simulink library "pidActiveLoad_lib"  (R2013a)
settings: Solver=ode45  StartTime=0.0  StopTime=10.0  RelTol=1e-3
undefined symbols (not defined in the file): dqActiveLoad, dqActiveLoad_lib, Ts
libraries: powerlib x8, simulink x3, breaker_lib x1, Load_lib x1, powerlib_meascontrol x1
settings Model: Creator=ed12083  LastModifiedBy=ed12083

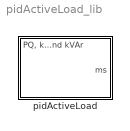
== system pidActiveLoad_lib ==
  pidActiveLoad : Subsystem  AncestorBlock=dqActiveLoad_lib/dqActiveLoad  mask{V=460}
      mask prompts: V "Vbus_RMS"

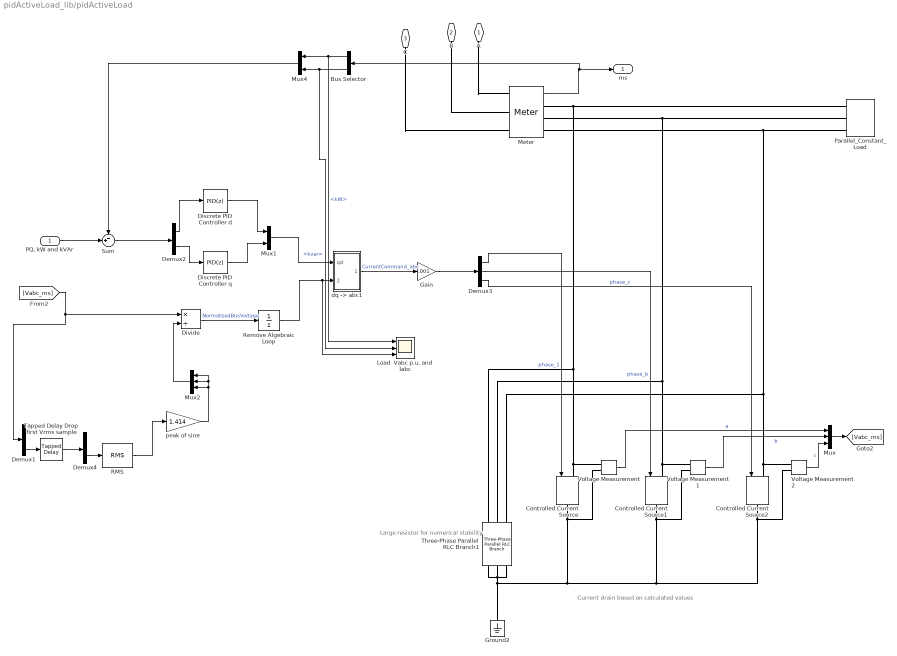
== system pidActiveLoad_lib/pidActiveLoad ==
  note: Current drain based on calculated values
  note: Large resistor for numerical stability
  "PQ, kW and kVAr" : Inport
  Bus Selector : BusSelector  OutputSignals=kW,kvar
  Controlled Current Source : powerlib/Electrical Sources/Controlled Current Source  Initialize=on  Source_Type=AC  Amplitude=0  Phase=0  Frequency=0  Measurements=None
  Controlled Current Source1 : powerlib/Electrical Sources/Controlled Current Source  Initialize=on  Source_Type=AC  Amplitude=0  Phase=0  Frequency=0  Measurements=None
  Controlled Current Source2 : powerlib/Electrical Sources/Controlled Current Source  Initialize=on  Source_Type=AC  Amplitude=0  Phase=0  Frequency=0  Measurements=None
  Demux1 : Demux  Outputs=3
  Demux2 : Demux  Outputs=2
  Demux3 : Demux  Outputs=3
  Demux4 : Demux  Outputs=2
  Discrete PID Controller d : simulink/Continuous/PID Controller  Controller=PID  TimeDomain=Discrete-time  SampleTime=Ts  IntegratorMethod=Forward Euler  FilterMethod=Forward Euler  Form=Parallel  P=0  I=2000  D=20  N=100  InitialConditionSource=internal  InitialConditionForIntegrator=0  InitialConditionForFilter=0  ExternalReset=none  LimitOutput=off  UpperSaturationLimit=inf  LowerSaturationLimit=-inf  LinearizeAsGain=off  AntiWindupMode=none  Kb=1  TrackingMode=off  Kt=1  PParamMin=[]  PParamMax=[]  IParamMin=[]  IParamMax=[]  DParamMin=[]  DParamMax=[]  NParamMin=[]  NParamMax=[]  KbParamMin=[]  KbParamMax=[]  KtParamMin=[]  KtParamMax=[]  POutMin=[]  POutMax=[]  IOutMin=[]  IOutMax=[]  DOutMin=[]  DOutMax=[]  NOutMin=[]  NOutMax=[]  KbOutMin=[]  KbOutMax=[]  KtOutMin=[]  KtOutMax=[]  IntegratorOutMin=[]  IntegratorOutMax=[]  FilterOutMin=[]  FilterOutMax=[]  SumOutMin=[]  SumOutMax=[]  SumI1OutMin=[]  SumI1OutMax=[]  SumI2OutMin=[]  SumI2OutMax=[]  SumI3OutMin=[]  SumI3OutMax=[]  SumDOutMin=[]  SumDOutMax=[]  SaturationOutMin=[]  SaturationOutMax=[]  IntegratorContinuousStateAttributes=''  IntegratorStateMustResolveToSignalObject=off  IntegratorRTWStateStorageClass=Auto  FilterContinuousStateAttributes=''  FilterStateMustResolveToSignalObject=off  FilterRTWStateStorageClass=Auto
  Discrete PID Controller q : simulink/Continuous/PID Controller  Controller=PID  TimeDomain=Discrete-time  SampleTime=Ts  IntegratorMethod=Forward Euler  FilterMethod=Forward Euler  Form=Parallel  P=0  I=-2000  D=-20  N=100  InitialConditionSource=internal  InitialConditionForIntegrator=0  InitialConditionForFilter=0  ExternalReset=none  LimitOutput=off  UpperSaturationLimit=inf  LowerSaturationLimit=-inf  LinearizeAsGain=off  AntiWindupMode=none  Kb=1  TrackingMode=off  Kt=1  PParamMin=[]  PParamMax=[]  IParamMin=[]  IParamMax=[]  DParamMin=[]  DParamMax=[]  NParamMin=[]  NParamMax=[]  KbParamMin=[]  KbParamMax=[]  KtParamMin=[]  KtParamMax=[]  POutMin=[]  POutMax=[]  IOutMin=[]  IOutMax=[]  DOutMin=[]  DOutMax=[]  NOutMin=[]  NOutMax=[]  KbOutMin=[]  KbOutMax=[]  KtOutMin=[]  KtOutMax=[]  IntegratorOutMin=[]  IntegratorOutMax=[]  FilterOutMin=[]  FilterOutMax=[]  SumOutMin=[]  SumOutMax=[]  SumI1OutMin=[]  SumI1OutMax=[]  SumI2OutMin=[]  SumI2OutMax=[]  SumI3OutMin=[]  SumI3OutMax=[]  SumDOutMin=[]  SumDOutMax=[]  SaturationOutMin=[]  SaturationOutMax=[]  IntegratorContinuousStateAttributes=''  IntegratorStateMustResolveToSignalObject=off  IntegratorRTWStateStorageClass=Auto  FilterContinuousStateAttributes=''  FilterStateMustResolveToSignalObject=off  FilterRTWStateStorageClass=Auto
  Divide : Product  Inputs=*/
  Gain : Gain  Gain=.001
  Ground2 : powerlib/Elements/Ground  LConnTagsString=a
  Load  Vabc p.u. and Iabc : Scope  NumInputPorts=3
      settings: ShowLegends=on  YMin=0~0~-1.5  YMax=800~175~1.5
  Meter : breaker_lib/Meter  Ts=Ts
  Mux : Mux  Inputs=3
  Mux1 : Mux  Inputs=2
  Mux2 : Mux  Inputs=3
  Mux4 : Mux  Inputs=2
  Parallel_Constant_Load : Load_lib/Parallel_Constant_Load  v=460  kVA=10  pf=.9
  RMS : powerlib_meascontrol/Measurements/RMS  TrueRMS=on  Freq=60  RMSInit=V/1.7321  Ts=0
  Remove Algebraic Loop : UnitDelay  SampleTime=-1
  Sum : Sum  Inputs=-+|
  Tapped Delay Drop first Vrms sample : simulink/Discrete/Tapped Delay  vinit=V/1.7321  samptime=-1  NumDelays=2  DelayOrder=Oldest  includeCurrent=off
  Three-Phase Parallel RLC Branch1 : powerlib/Elements/Three-Phase Parallel RLC Branch  LConnTagsString=A|B|C  RConnTagsString=A|B|C  BranchType=RLC  Resistance=1e6  Inductance=inf  Capacitance=0  Measurements=None
  Voltage Measurement : powerlib/Measurements/Voltage Measurement  PhasorSimulation=off  OutputType=Complex  PSBequivalent=0
  Voltage Measurement1 : powerlib/Measurements/Voltage Measurement  PhasorSimulation=off  OutputType=Complex  PSBequivalent=0
  Voltage Measurement2 : powerlib/Measurements/Voltage Measurement  PhasorSimulation=off  OutputType=Complex  PSBequivalent=0
  "dq -> abc1" : Subsystem
  peak of sine : Gain  Gain=1.414
  A : PMIOPort  Port=1  Side=Left
  B : PMIOPort  Port=2  Side=Left
  C : PMIOPort  Port=3  Side=Left
  ms : Outport
  wires:
  Mux4/1 -> Sum/1
  Gain/1 -> Demux3/1
  Remove Algebraic Loop/1 -> "dq -> abc1"/2(Vabc), Load  Vabc p.u. and Iabc/3
  Discrete PID Controller q/1 -> Mux1/2
  Discrete PID Controller d/1 -> Mux1/1
  Mux1/1 -> "dq -> abc1"/1(qd)
  Demux2/2 -> Discrete PID Controller q/1
  Demux2/1 -> Discrete PID Controller d/1
  Sum/1 -> Demux2/1
  "dq -> abc1"/1(abc) -> Gain/1  "CurrentCommand_abc"
  Bus Selector/1 -> Mux4/1, Load  Vabc p.u. and Iabc/1  "<kW>"
  Bus Selector/2 -> Mux4/2, Load  Vabc p.u. and Iabc/2  "<kvar>"
  Demux4/2 -> RMS/1
  Demux1/3 -> Tapped Delay Drop first Vrms sample/1
  Tapped Delay Drop first Vrms sample/1 -> Demux4/1
  [Vabc_ms] -> Demux1/1, Divide/1
  Mux2/1 -> Divide/2
  peak of sine/1 -> Mux2/3, Mux2/2, Mux2/1
  RMS/1 -> peak of sine/1
  Demux3/3 -> Controlled Current Source2/1  "phase_c"
  Voltage Measurement1/1 -> Mux/2  "b"
  Mux/1 -> [Vabc_ms]
  Demux3/1 -> Controlled Current Source/1  "phase_1"
  Meter/1 -> ms/1, Bus Selector/1
  Demux3/2 -> Controlled Current Source1/1  "phase_b"
  Voltage Measurement/1 -> Mux/1  "a"
  Voltage Measurement2/1 -> Mux/3  "c"
  "PQ, kW and kVAr"/1 -> Sum/2
  Divide/1 -> Remove Algebraic Loop/1  "NormalizedBusVoltage"
  connections:
  A/RConn1 -- Meter/LConn1
  B/RConn1 -- Meter/LConn2
  C/RConn1 -- Meter/LConn3
  Controlled Current Source1/LConn1 -- Parallel_Constant_Load/RConn2 -- Meter/RConn2 -- Three-Phase Parallel RLC Branch1/RConn2 -- Voltage Measurement1/LConn1
  Controlled Current Source/LConn1 -- Meter/RConn1 -- Parallel_Constant_Load/RConn1 -- Three-Phase Parallel RLC Branch1/RConn1 -- Voltage Measurement/LConn1
  Controlled Current Source2/LConn1 -- Parallel_Constant_Load/RConn3 -- Meter/RConn3 -- Three-Phase Parallel RLC Branch1/RConn3 -- Voltage Measurement2/LConn1
  Controlled Current Source2/RConn1 -- Three-Phase Parallel RLC Branch1/LConn1 -- Three-Phase Parallel RLC Branch1/LConn2 -- Three-Phase Parallel RLC Branch1/LConn3 -- Ground2/LConn1 -- Voltage Measurement/LConn2 -- Controlled Current Source/RConn1 -- Voltage Measurement1/LConn2 -- Controlled Current Source1/RConn1 -- Voltage Measurement2/LConn2

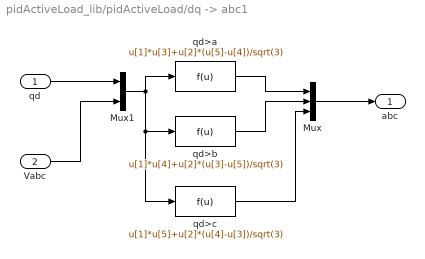
== system pidActiveLoad_lib/pidActiveLoad/dq -> abc1 ==
  qd : Inport  OutDataTypeStr=double  PortDimensions=2
  Vabc : Inport  Port=2  PortDimensions=3
  Mux : Mux  Inputs=3
  Mux1 : Mux  Inputs=2
  qd>a : Fcn  Expr=u[1]*u[3]+u[2]*(u[5]-u[4])/sqrt(3)
  qd>b : Fcn  Expr=u[1]*u[4]+u[2]*(u[3]-u[5])/sqrt(3)
  qd>c : Fcn  Expr=u[1]*u[5]+u[2]*(u[4]-u[3])/sqrt(3)
  abc : Outport  OutDataTypeStr=double  PortDimensions=3
  wires:
  qd>b/1 -> Mux/2
  qd/1 -> Mux1/1
  qd>c/1 -> Mux/3
  Mux1/1 -> qd>c/1, qd>b/1, qd>a/1
  qd>a/1 -> Mux/1
  Vabc/1 -> Mux1/2
  Mux/1 -> abc/1
